simulink model "simulator1D"  (R2025b)
settings: Solver=VariableStepAuto  StartTime=0.0  StopTime=100  FixedStep=1e-4  RelTol=1e-3
values from neighbouring files (symbols this model uses):
  x1_0 = xL0+q1_rot*[0;0;L1]    [parametrosCarga4x.m]
settings Model: Creator=ateveraz  LastModifiedBy=ateveraz

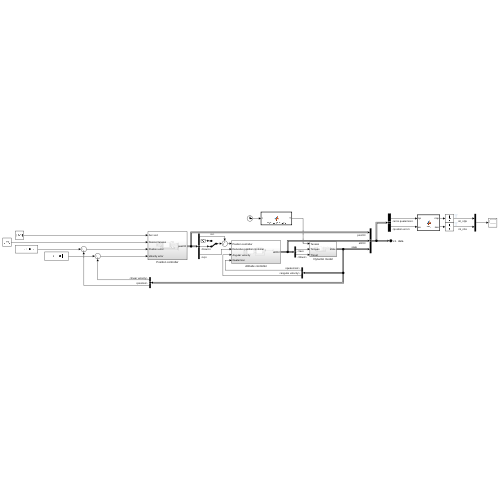
[thumbnail: Simulink's stored preview of the top-level diagram]
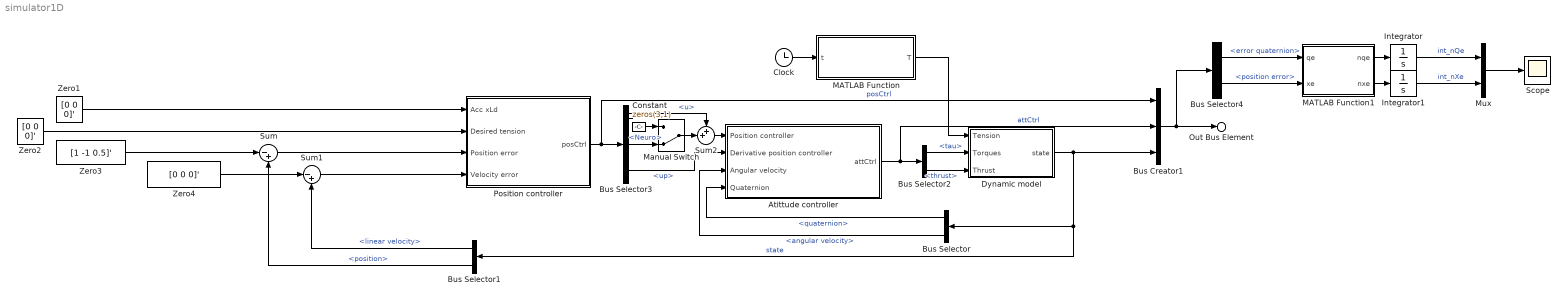
== system simulator1D ==
  Atittude controller : Subsystem
  Bus Creator1 : BusCreator  Inputs=3
  Bus Selector : BusSelector  OutputSignals=quaternion,angular velocity
  Bus Selector1 : BusSelector  OutputSignals=linear velocity,position
  Bus Selector2 : BusSelector  OutputSignals=tau,thrust
  Bus Selector3 : BusSelector  OutputSignals=u,Neuro,up
  Bus Selector4 : BusSelector  OutputSignals=attCtrl.error quaternion,posCtrl.position error
  Clock : Clock
  Constant : Constant  Value=zeros(3,1)
  Dynamic model : Subsystem
  Integrator : Integrator
  Integrator1 : Integrator
  MATLAB Function : MATLAB Function  TreatAsAtomicUnit=on
  MATLAB Function1 : MATLAB Function  TreatAsAtomicUnit=on
  Manual Switch : ManualSwitch  CurrentSetting=0
  Mux : Mux  Inputs=2
  Position controller : Subsystem
  Scope : Scope
      settings: ActiveDisplayYMinimum=-0.40133552260811456  ActiveDisplayYMaximum=3.6120197034730319
  Sum : Sum  Inputs=|-+
  Sum1 : Sum  Inputs=|-+
  Sum2 : Sum  Inputs=++|
  Zero1 : Constant  Value=[0 0 0]'  OutDataTypeStr=Inherit: Inherit via back propagation
  Zero2 : Constant  Value=[0 0 0]'  OutDataTypeStr=Inherit: Inherit via back propagation
  Zero3 : Constant  Value=[1 -1 0.5]'  OutDataTypeStr=Inherit: Inherit via back propagation
  Zero4 : Constant  Value=[0 0 0]'  OutDataTypeStr=Inherit: Inherit via back propagation
  Out Bus Element : Outport  PortName=x1  Element=data
  wires:
  Position controller/1(posCtrl) -> Bus Creator1/1, Bus Selector3/1  "posCtrl"
  Atittude controller/1(attCtrl) -> Bus Creator1/2, Bus Selector2/1  "attCtrl"
  Dynamic model/1(state) -> Bus Selector/1, Bus Selector1/1, Bus Creator1/3  "state"
  Bus Creator1/1 -> Bus Selector4/1, Out Bus Element/1
  MATLAB Function/1(T) -> Dynamic model/1(Tension)
  Bus Selector3/3 -> Atittude controller/2(Derivative position controller)  "<up>"
  Bus Selector1/1 -> Sum1/2  "<linear velocity>"
  Zero3/1 -> Sum/1
  Bus Selector2/2 -> Dynamic model/3(Thrust)  "<thrust>"
  Bus Selector1/2 -> Sum/2  "<position>"
  Bus Selector/1 -> Atittude controller/4(Quaternion)  "<quaternion>"
  Sum/1 -> Position controller/3(Position error)
  Zero1/1 -> Position controller/1(Acc xLd)
  Zero2/1 -> Position controller/2(Desired tension)
  Bus Selector2/1 -> Dynamic model/2(Torques)  "<tau>"
  Bus Selector3/1 -> Sum2/1  "<u>"
  Zero4/1 -> Sum1/1
  Bus Selector/2 -> Atittude controller/3(Angular velocity)  "<angular velocity>"
  Sum1/1 -> Position controller/4(Velocity error)
  Clock/1 -> MATLAB Function/1(t)
  Sum2/1 -> Atittude controller/1(Position controller)
  Bus Selector3/2 -> Manual Switch/2  "<Neuro>"
  Bus Selector4/1 -> MATLAB Function1/1(qe)  "<error quaternion>"
  Bus Selector4/2 -> MATLAB Function1/2(xe)  "<position error>"
  MATLAB Function1/1(nqe) -> Integrator/1
  MATLAB Function1/2(nxe) -> Integrator1/1
  Integrator/1 -> Mux/1  "int_nQe"
  Mux/1 -> Scope/1
  Integrator1/1 -> Mux/2  "int_nXe"
  Manual Switch/1 -> Sum2/2
  Constant/1 -> Manual Switch/1

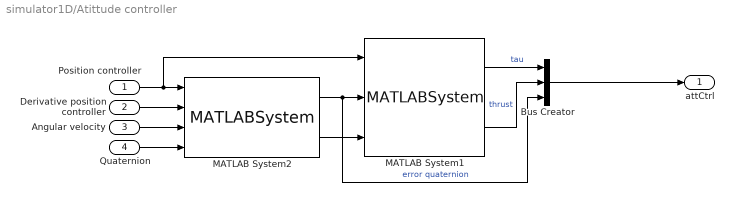
== system simulator1D/Atittude controller ==
  Position controller : Inport
  Derivative position controller : Inport  Port=2
  Angular velocity : Inport  Port=3
  Quaternion : Inport  Port=4
  Bus Creator : BusCreator  Inputs=3
  MATLAB System1 : MATLABSystem  System=AttitudeController  Kd=2.0  beta=0.5  gamma=1.0  rho=5.0  SimulateUsing=Code generation
      mask Type: AttitudeController
  MATLAB System2 : MATLABSystem  System=DesiredAttitude  SimulateUsing=Code generation
      mask Type: DesiredAttitude
  attCtrl : Outport
  wires:
  Angular velocity/1 -> MATLAB System2/3
  MATLAB System2/2 -> MATLAB System1/3
  Position controller/1 -> MATLAB System1/1, MATLAB System2/1
  Quaternion/1 -> MATLAB System2/4
  MATLAB System2/1 -> Bus Creator/3, MATLAB System1/2  "error quaternion"
  Derivative position controller/1 -> MATLAB System2/2
  MATLAB System1/2 -> Bus Creator/2  "thrust"
  Bus Creator/1 -> attCtrl/1
  MATLAB System1/1 -> Bus Creator/1  "tau"

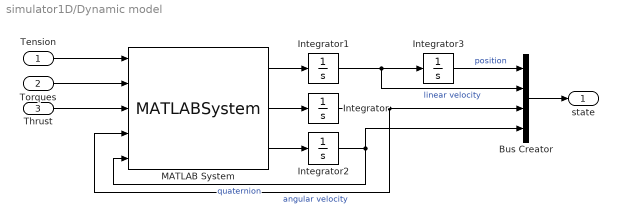
== system simulator1D/Dynamic model ==
  Tension : Inport
  Torques : Inport  Port=2
  Thrust : Inport  Port=3
  Bus Creator : BusCreator  Inputs=4
  Integrator : Integrator  InitialCondition=[0 0 0]'
  Integrator1 : Integrator  InitialCondition=[0 0 0]'
  Integrator2 : Integrator  InitialCondition=[1 0 0 0]'
  Integrator3 : Integrator  InitialCondition=x1_0
  MATLAB System : MATLABSystem  System=Modelx4  mass=0.4  inertia_matrix=[ 2.098e3, 63.577538, -2.002648; 63.577538, 2.102e3, 0.286186; -2.002648, 0.286186, 4.068e3 ] * 1e-6  SimulateUsing=Code generation
      mask Type: Modelx4
  state : Outport
  wires:
  MATLAB System/1 -> Integrator1/1
  Integrator3/1 -> Bus Creator/1  "position"
  MATLAB System/3 -> Integrator2/1
  MATLAB System/2 -> Integrator/1
  Integrator2/1 -> MATLAB System/5, Bus Creator/4  "quaternion"
  Torques/1 -> MATLAB System/2
  Integrator1/1 -> Bus Creator/2, Integrator3/1  "linear velocity"
  Thrust/1 -> MATLAB System/3
  Integrator/1 -> MATLAB System/4, Bus Creator/3  "angular velocity"
  Bus Creator/1 -> state/1
  Tension/1 -> MATLAB System/1

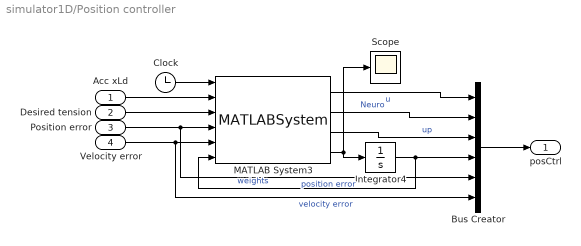
== system simulator1D/Position controller ==
  Acc xLd : Inport
  Desired tension : Inport  Port=2
  Position error : Inport  Port=3
  Velocity error : Inport  Port=4
  Bus Creator : BusCreator  Inputs=6
  Clock : Clock
  Integrator4 : Integrator  InitialCondition=zeros(3,15)
  MATLAB System3 : MATLABSystem  System=PositionController  Kd=diag([2 2 2])  alpha=0.8  mass=0.4  Gamma=0.3  kappa=20  k=5  N_neurons=15  center_range=0.5  eta_width=linspace(1,10,15)  SimulateUsing=Interpreted execution
      mask Type: PositionController
  Scope : Scope
      settings: ActiveDisplayYMinimum=-0.3136708420360429  ActiveDisplayYMaximum=1.3671797342518703
  posCtrl : Outport
  wires:
  Position error/1 -> Bus Creator/5, MATLAB System3/4  "position error"
  Acc xLd/1 -> MATLAB System3/2
  Integrator4/1 -> MATLAB System3/6, Bus Creator/4  "weights"
  Bus Creator/1 -> posCtrl/1
  Velocity error/1 -> Bus Creator/6, MATLAB System3/5  "velocity error"
  MATLAB System3/4 -> Integrator4/1, Scope/1
  Desired tension/1 -> MATLAB System3/3
  MATLAB System3/1 -> Bus Creator/1  "u"
  MATLAB System3/2 -> Bus Creator/2  "Neuro"
  MATLAB System3/3 -> Bus Creator/3  "up"
  Clock/1 -> MATLAB System3/1

== matlab function simulator1D/MATLAB Function ==
  data: t input; T output
function T = virtualTension(t)
    T = zeros(3,1);

    if (t > 20 && t < 30)
        a = 0.1;
        T(1) = a * cos(t-20);
        T(2) = -a * sin(t-20);
        T(3) = a * cos(2*t);
    end
end

== matlab function simulator1D/MATLAB Function1 ==
  data: qe input; nqe output; xe input; nxe output
function [nqe, nxe] = fcn(qe,xe)
    nqe = norm(qe(2:4));
    nxe = norm(xe);
end
